simulink model "RAMP"  (R2018b)
settings: Solver=FixedStepDiscrete  StartTime=0.0  StopTime=10.0  FixedStep=1e-4  RelTol=1e-3
settings Model: Creator=F001456D  LastModifiedBy=C000874D
settings DebuggingCC: InheritedTsInSrcMsg=none  RootOutportRequireBusObject=error  StrictBusMsg=ErrorOnBusTreatedAsVector
settings HardwareCC: ProdBitPerPointer=32  ProdBitPerSizeT=32  ProdBitPerPtrDiffT=32  ProdLargestAtomicInteger=Long  ProdWordSize=32  ProdHWDeviceType=ARM Compatible->ARM 7
settings SFSimCC: SimUseLocalCustomCode=off
settings RTWCC: SystemTargetFile=MTRealTime_ZYNQ.tlc  TemplateMakefile=MTRealTime_ZYNQ.tmf  Description=MT RealTime ZYNQ Target  RTWUseLocalCustomCode=off
settings CodeAppCC: StateflowObjectComments=on
settings STFCustomTargetCC: TargetLangStandard=C99 (ISO)  GRTInterface=on  SystemTargetFile=MTRealTime_ZYNQ.tlc
settings GRTTargetCC: ParMdlRefBuildCompliant=off  CompOptLevelCompliant=off  ConcurrentExecutionCompliant=off  CombineOutputUpdateFcns=off  MatFileLogging=off  CPPClassGenCompliant=off  GRTInterface=on  UseToolchainInfoCompliant=off
settings SimscapeCC: SimscapeNormalizeSystem=off

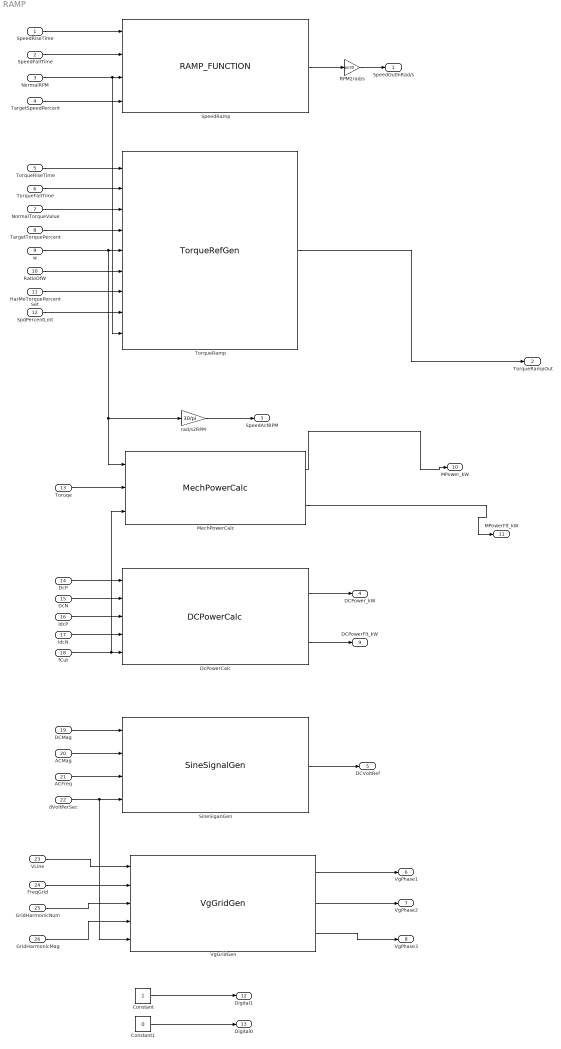
== system RAMP ==
  SpeedRiseTime : Inport
  SpeedFallTime : Inport  Port=2
  NormalRPM : Inport  Port=3
  TargetSpeedPercent : Inport  Port=4
  TorqueRiseTime : Inport  Port=5
  TorqueFallTime : Inport  Port=6
  NormalTorqueValue : Inport  Port=7
  TargetTorquePercent : Inport  Port=8
  w : Inport  Port=9
  RatioOfW : Inport  Port=10
  HarMoTorquePercentSet : Inport  Port=11
  SpdPercentLmt : Inport  Port=12
  Toruqe : Inport  Port=13
  DcP : Inport  Port=14
  DcN : Inport  Port=15
  IdcP : Inport  Port=16
  IdcN : Inport  Port=17
  fCut : Inport  Port=18
  DCMag : Inport  Port=19
  ACMag : Inport  Port=20
  ACFreq : Inport  Port=21
  dVoltPerSec : Inport  Port=22
  VLine : Inport  Port=23
  FreqGrid : Inport  Port=24
  GridHarmonicNum : Inport  Port=25
  GridHarmonicMag : Inport  Port=26
  Constant : Constant
  Constant1 : Constant  Value=0
  DcPowerCalc : S-Function  InitFcn=try, set_param(gcb,'FunctionName','DCPowerCalc'), end  FunctionName=DCPowerCalc  SFunctionModules=DCPowerCalc_wrapper  SFunctionDeploymentMode=off  EnableBusSupport=off  mask(S-Function Builder){}
      mask help: Simulink:masks:SFunctionBuilder_MD
      mask init:
      | val = [[.9  0.75 0.75 1 1 .9 .9 1]',[1 1 0.75 0.75 .9 .9 1 .9]'];try , sys = get_param(gcb,'SfunBuilderFcnName');if isempty(sys), sys = get_param(gcb,'FunctionName'); end,catch, sys = get_param(gcb,'FunctionName'); end
      settings: CopyFcn=set_param(gcbh,'LinkStatus','none')  PreSaveFcn=try, set_param(gcb,'FunctionName','DCPowerCalc'), end  OpenFcn=sfunctionwizard(gcbh)
      mask Display: plot(val(:,1),val(:,2)),disp(sys), port_label('input',1,'VdcP'), port_label('input',2,'VdcN'), port_label('input',3,'IdcP'), port_label('input',4,'IdcN'), port_label('input',5,'fCut'), port_label('output',1,'DCPower_kW'), port_label('output',2,'DCPowerFlt_kW')
  MechPowerCalc : S-Function  InitFcn=try, set_param(gcb,'FunctionName','MechPowerCalc'), end  FunctionName=MechPowerCalc  SFunctionModules=MechPowerCalc_wrapper  SFunctionDeploymentMode=off  EnableBusSupport=off  mask(S-Function Builder){}
      mask help: Simulink:masks:SFunctionBuilder_MD
      mask init: same as RAMP/DcPowerCalc
      settings: CopyFcn=set_param(gcbh,'LinkStatus','none')  PreSaveFcn=try, set_param(gcb,'FunctionName','MechPowerCalc'), end  OpenFcn=sfunctionwizard(gcbh)
      mask Display: plot(val(:,1),val(:,2)),disp(sys), port_label('input',1,'Wm'), port_label('input',2,'Torque'), port_label('input',3,'fCut'), port_label('output',1,'MechPower_kW'), port_label('output',2,'MechPowerFlt_kW')
  RPM2rad/s : Gain  Gain=pi/30
  SineSiganGen : S-Function  InitFcn=try, set_param(gcb,'FunctionName','SineSignalGen'), end  FunctionName=SineSignalGen  SFunctionModules=SineSignalGen_wrapper  SFunctionDeploymentMode=off  EnableBusSupport=off  mask(S-Function Builder){}
      mask help: Simulink:masks:SFunctionBuilder_MD
      mask init: same as RAMP/DcPowerCalc
      settings: CopyFcn=set_param(gcbh,'LinkStatus','none')  PreSaveFcn=try, set_param(gcb,'FunctionName','SineSignalGen'), end  OpenFcn=sfunctionwizard(gcbh)
      mask Display: plot(val(:,1),val(:,2)),disp(sys), port_label('input',1,'DCMag'), port_label('input',2,'ACMag'), port_label('input',3,'Freq'), port_label('input',4,'dVoltPerSec'), port_label('output',1,'SineOut')
  SpeedRamp : S-Function  InitFcn=try, set_param(gcb,'FunctionName','RAMP_FUNCTION'), end  FunctionName=RAMP_FUNCTION  SFunctionModules=RAMP_FUNCTION_wrapper  SFunctionDeploymentMode=off  EnableBusSupport=off  mask(S-Function Builder){}
      mask help: Simulink:masks:SFunctionBuilder_MD
      mask init: same as RAMP/DcPowerCalc
      settings: CopyFcn=set_param(gcbh,'LinkStatus','none')  PreSaveFcn=try, set_param(gcb,'FunctionName','RAMP_FUNCTION'), end  OpenFcn=sfunctionwizard(gcbh)
      mask Display: plot(val(:,1),val(:,2)),disp(sys), port_label('input',1,'RiseTime'), port_label('input',2,'FallTime'), port_label('input',3,'NormalValue'), port_label('input',4,'DestValueRatio'), port_label('output',1,'RampOut')
  TorqueRamp : S-Function  InitFcn=try, set_param(gcb,'FunctionName','TorqueRefGen'), end  FunctionName=TorqueRefGen  SFunctionModules=TorqueRefGen_wrapper  SFunctionDeploymentMode=off  EnableBusSupport=off  mask(S-Function Builder){}
      mask help: Simulink:masks:SFunctionBuilder_MD
      mask init: same as RAMP/DcPowerCalc
      settings: CopyFcn=set_param(gcbh,'LinkStatus','none')  PreSaveFcn=try, set_param(gcb,'FunctionName','TorqueRefGen'), end  OpenFcn=sfunctionwizard(gcbh)
      mask Display: plot(val(:,1),val(:,2)),disp(sys), port_label('input',1,'RiseTime'), port_label('input',2,'FallTime'), port_label('input',3,'NormalValue'), port_label('input',4,'DestValuePercent'), port_label('input',5,'w'), port_label('input',6,'RatioOfW'), port_label('input',7,'HarmoTorquePercent'), port_label('input',8,'SpdPercentLmt'), port_label('input',9,'RPMNorm'), port_label('output',1,'RampOut')
  VgGridGen : S-Function  InitFcn=try, set_param(gcb,'FunctionName','VgGridGen'), end  FunctionName=VgGridGen  SFunctionModules=VgGridGen_wrapper  SFunctionDeploymentMode=off  EnableBusSupport=off  mask(S-Function Builder){}
      mask help: Simulink:masks:SFunctionBuilder_MD
      mask init: same as RAMP/DcPowerCalc
      settings: CopyFcn=set_param(gcbh,'LinkStatus','none')  PreSaveFcn=try, set_param(gcb,'FunctionName','VgGridGen'), end  OpenFcn=sfunctionwizard(gcbh)
      mask Display: plot(val(:,1),val(:,2)),disp(sys), port_label('input',1,'ACLine'), port_label('input',2,'Freq'), port_label('input',3,'HarmonicNum'), port_label('input',4,'HarmonicMag'), port_label('input',5,'dVoltPerSec'), port_label('output',1,'VgPhaseA'), port_label('output',2,'VgPhaseB'), port_label('output',3,'VgPhaseC')
  rad/s2RPM : Gain  Gain=30/pi
  SpeedOutInRad/s : Outport
  TorqueRampOut : Outport  Port=2
  SpeedActRPM : Outport  Port=3
  DCPower_kW : Outport  Port=4
  DCVoltRef : Outport  Port=5
  VgPhase1 : Outport  Port=6
  VgPhase2 : Outport  Port=7
  VgPhase3 : Outport  Port=8
  DCPowerFlt_kW : Outport  Port=9
  MPower_kW : Outport  Port=10
  MPowerFlt_kW : Outport  Port=11
  Digital1 : Outport  Port=12
  Digital0 : Outport  Port=13
  wires:
  SpeedRiseTime/1 -> SpeedRamp/1
  SpeedFallTime/1 -> SpeedRamp/2
  TargetSpeedPercent/1 -> SpeedRamp/4
  NormalRPM/1 -> TorqueRamp/9, SpeedRamp/3
  SineSiganGen/1 -> DCVoltRef/1
  SpeedRamp/1 -> RPM2rad/s/1
  RPM2rad/s/1 -> SpeedOutInRad/s/1
  rad/s2RPM/1 -> SpeedActRPM/1
  DcP/1 -> DcPowerCalc/1
  DcN/1 -> DcPowerCalc/2
  IdcP/1 -> DcPowerCalc/3
  IdcN/1 -> DcPowerCalc/4
  fCut/1 -> MechPowerCalc/3, DcPowerCalc/5
  DcPowerCalc/1 -> DCPower_kW/1
  Toruqe/1 -> MechPowerCalc/2
  DCMag/1 -> SineSiganGen/1
  ACMag/1 -> SineSiganGen/2
  ACFreq/1 -> SineSiganGen/3
  dVoltPerSec/1 -> VgGridGen/5, SineSiganGen/4
  SpdPercentLmt/1 -> TorqueRamp/8
  TorqueRiseTime/1 -> TorqueRamp/1
  w/1 -> TorqueRamp/5, MechPowerCalc/1, rad/s2RPM/1
  HarMoTorquePercentSet/1 -> TorqueRamp/7
  TargetTorquePercent/1 -> TorqueRamp/4
  RatioOfW/1 -> TorqueRamp/6
  TorqueFallTime/1 -> TorqueRamp/2
  NormalTorqueValue/1 -> TorqueRamp/3
  TorqueRamp/1 -> TorqueRampOut/1
  GridHarmonicMag/1 -> VgGridGen/4
  VgGridGen/2 -> VgPhase2/1
  VLine/1 -> VgGridGen/1
  FreqGrid/1 -> VgGridGen/2
  GridHarmonicNum/1 -> VgGridGen/3
  VgGridGen/3 -> VgPhase3/1
  VgGridGen/1 -> VgPhase1/1
  DcPowerCalc/2 -> DCPowerFlt_kW/1
  MechPowerCalc/2 -> MPowerFlt_kW/1
  MechPowerCalc/1 -> MPower_kW/1
  Constant/1 -> Digital1/1
  Constant1/1 -> Digital0/1
